simulink model "FactorialCalc_SF_Topic3_Task2"  (R2019a)
settings: Solver=FixedStepDiscrete  StartTime=0.0  StopTime=10.0  RelTol=1e-3
settings Model: Creator=Raouf  LastModifiedBy=Raouf
settings OptimizationCC: DefaultParameterBehavior=Inlined  EnhancedBackFolding=on  PassReuseOutputArgsAs=Individual arguments  OptimizeBlockOrder=speed  DifferentSizesBufferReuse=on  OptimizationCustomize=off
settings DebuggingCC: ParameterTunabilityLossMsg=error
settings SFSimCC: MATLABDynamicMemAlloc=off
settings RTWCC: SystemTargetFile=ert.tlc  GenCodeOnly=on  TemplateMakefile=ert_default_tmf  GenerateReport=on  IncludeHyperlinkInReport=on  LaunchReport=on  GenerateTraceInfo=on  GenerateTraceReport=on  GenerateTraceReportSl=on  GenerateTraceReportSf=on  GenerateTraceReportEml=on
settings CodeAppCC: ForceParamTrailComments=on  IgnoreCustomStorageClasses=off  OperatorAnnotations=on  SimulinkDataObjDesc=on  SFDataObjDesc=on  InsertBlockDesc=on
settings ERTTargetCC: TargetLangStandard=C99 (ISO)  GenerateSampleERTMain=on  InlinedParameterPlacement=NonHierarchical  ERTCustomFileTemplate=example_file_process.tlc

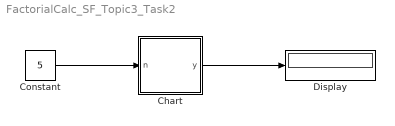
== system FactorialCalc_SF_Topic3_Task2 ==
  Chart : Stateflow chart  TreatAsAtomicUnit=on
  Constant : Constant  Value=5  OutDataTypeStr=uint32
  Display : Display
  wires:
  Chart/1(y) -> Display/1
  Constant/1 -> Chart/1(n)

== stateflow chart FactorialCalc_SF_Topic3_Task2/Chart ==
  (default) -> (junction 1) : {  y = 1;
      |    u = n;  }
  (junction 3) -> (junction 1) [order 1] : [u > 1]
  (junction 1) -> (junction 3) : {  y = y*u;
      |    u = u-1;  }
  (junction 3) -> (junction 12) [order 2]
  data: y output uint32; n input uint32; u local uint32
